simulink model "CarsimOut_1210"  (R2015b)
settings: Solver=VariableStepAuto  StartTime=0.0  StopTime=10.0  RelTol=1e-3
undefined symbols (not defined in the file or in its folder): sigbuilder_block
libraries: Solver_SF x2
settings Model: Creator=ASUS  LastModifiedBy=ASUS

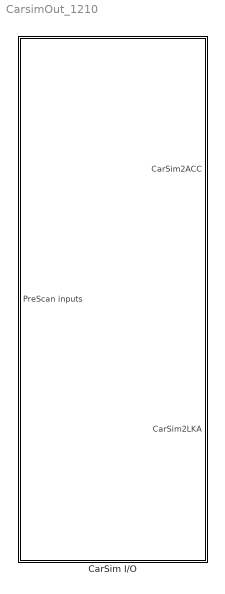
== system CarsimOut_1210 ==
  CarSim I/O : Subsystem

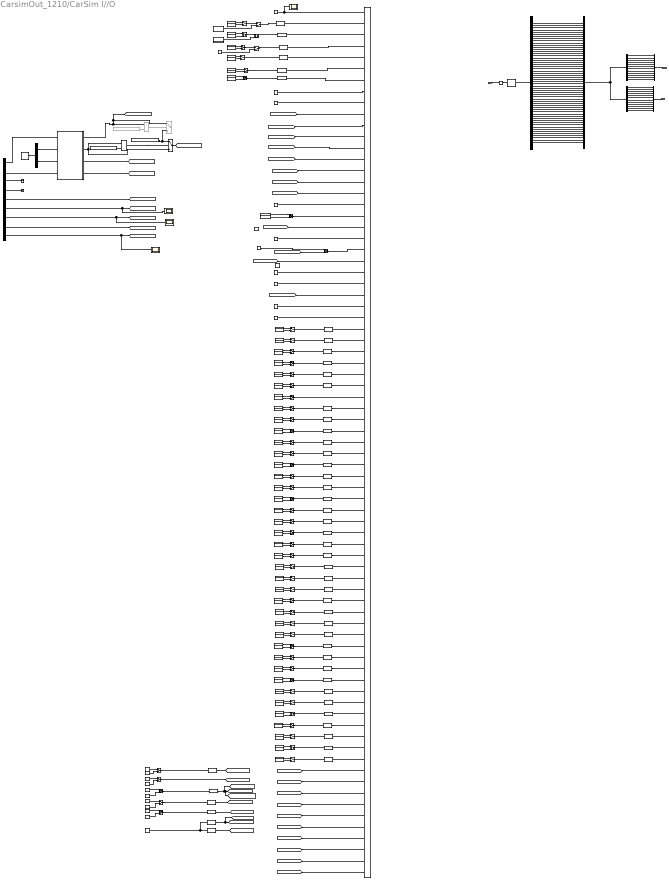
== system CarsimOut_1210/CarSim I//O ==
  PreScan inputs : Inport
  AccelActuPosHSC1_d : Constant  Value=0.31  OutDataTypeStr=double
      settings: AttributesFormatString=%<DataType=%<OutDataTypeStr>>
  BrkPdlPos_H1HSC1_d : Constant  Value=0  OutDataTypeStr=double
  Bus Creator : BusCreator  Inputs=77
  Bus Creator1 : BusCreator  Inputs=56
  Bus Creator2 : BusCreator  Inputs=12
  Bus Creator3 : BusCreator  Inputs=12
  Bus Selector : BusSelector  OutputSignals=EnSpdHSC1_d[rpm] (signal 36),EnToqActuExtdRngHSC1_d[N M] (signal 37),WhlGndVelRDrvn_H1HSC2_d[km/h] (signal 38),WhlGndVelLDrvn_H1HSC2_d[km/h] (signal 39),WhlGndVelRNonDrvn_H1HSC2_d[km/h] (signal 40),WhlGndVelLNonDrvn_H1HSC2_d[km/h] (signal 41),VSELongtAcc_H1HSC1_d[g] (signal 42),VehDynYawRate_H1HSC1_d[deg/s] (signal 43),StrgWhlAngGrd_HSC2_d[deg/s] (signal 44),SteeringWheelAngle[deg] (signal 34),AccelActuPosHSC1_d (signal 45),AccelEfctvPosHSC1_d (signal 46)
  Bus Selector1 : BusSelector  OutputSignals=VehicleCoG_Vx[km/h] (signal 4),Mz_Kp_L1[NM] (signal 48),Mz_Kp_L1[NM] (signal 49),Steer_L1[deg] (signal 50),Steer_R1[deg] (signal 51),F_TRdL1[N] (signal 52),F_TRdR1[N] (signal 53),SteeringWheelAngle[deg] (signal 34),VehDynYawRate_H1HSC1_d[deg/s] (signal 43),Ax_SM[g] (signal 54),Ay_SM[g] (signal 55),GearStatus (signal 56)
  CarSim S-Function2 : Solver_SF/CarSim S-Function2  Priority=1  VehicleCode=i_i  SIMFILE=simfile.sim
      settings: AttributesFormatString=Vehicle Code: %<VehicleCode>
  Carsim Trans Module : Subsystem
  Constant1 : Constant  Value=100
  Constant{2..3,5,8,10,13,16,18,20..21,23,26..27,29,31..32,34,38,40..41,43,45..46,48,52..53,55,58,60..61,63,66,68..69,71,74..75,77,80,82..83,85,88..89} (44 alike) : Constant  Value=0
  Constant{4,6..7,9,11..12,14,17,22,24,28,30,33,35..37,39,42,44,47,49..51,54,56..57,59,62,64..65,67,70,72..73,76,78..79,81,84,86..87,90..91} (43 alike) : Constant
  Constant15 : Constant  OutDataTypeStr=uint8
  Constant19 : Constant  Value=-100
  Constant25 : Constant  Value=300
  DA_IN_DgrObjSyncCtr_u8 : Constant  Value=0  OutDataTypeStr=uint8
  Data Type Conversion{,1..5,10,17,25,32,49,52} (12 alike) : DataTypeConversion  OutDataTypeStr=uint8
  Data Type Conversion{6..8,11..16,18..24,26..31,33..38} (28 alike) : DataTypeConversion
  Data Type Conversion{39..44} (6 alike) : DataTypeConversion  OutDataTypeStr=boolean
  Data Type Conversion{50..51,53..54} (4 alike) : DataTypeConversion  OutDataTypeStr=single
  Demux : Demux  Outputs=56
  Demux1 : Demux  Outputs=[1 3]
  Demux2 : Demux  Outputs=[1 3 1 1 1 1 1 1 1]
  DrvrSbltAtcHSC1_u8 : Constant  OutDataTypeStr=uint8
  EPBAppcnStsHSC1_u8 : Constant  Value=0  OutDataTypeStr=uint8
  EnTypHSC2_u8 : Constant  OutDataTypeStr=uint8
  FntLatDist1 : Constant  Value=3  OutDataTypeStr=double
      settings: AttributesFormatString=%<OutDataTypeStr>
  FntLatDist2 : Constant  Value=0  OutDataTypeStr=double
      settings: AttributesFormatString=%<OutDataTypeStr>
  FntLatDist3 : Constant  OutDataTypeStr=double
      settings: AttributesFormatString=%<OutDataTypeStr>
  FntLatDist4 : Constant  Value=0  OutDataTypeStr=double
      settings: AttributesFormatString=%<OutDataTypeStr>
  FntLatDist5 : Constant  Value=13  OutDataTypeStr=double
      settings: AttributesFormatString=%<OutDataTypeStr>
  FntLatDist6 : Constant  Value=0  OutDataTypeStr=double
      settings: AttributesFormatString=%<OutDataTypeStr>
  ID_LOCKON_u1 : Constant  Value=5  OutDataTypeStr=uint8
  ID_LOCKON_u2 : Constant  Value=0  OutDataTypeStr=uint8
  ID_LOCKON_u3 : Constant  Value=5  OutDataTypeStr=uint8
  ID_LOCKON_u4 : Constant  Value=0  OutDataTypeStr=uint8
  ID_LOCKON_u8 : Constant  Value=5  OutDataTypeStr=uint8
  Lead Car : Solver_SF/CarSim S-Function2  Priority=1  VehicleCode=i_i  SIMFILE=Radar_Acc_ExtSen_Car_1.sim
      settings: AttributesFormatString=Vehicle Code: %<VehicleCode>
  Manual Switch{1,7,11,14,48..49,55} (7 alike) : ManualSwitch  CurrentSetting=0
  Manual Switch{2..6,8..10,12..13,15..47,50..54} (48 alike) : ManualSwitch
  Memory : Memory
  PtBrkPdlDscrtInptStsHSC1_u8 : Constant  Value=0  OutDataTypeStr=uint8
  Pulse Generator : DiscretePulseGenerator  PulseType=Time based  Period=100  PulseWidth=5  PhaseDelay=0.1
  Relational Operator2 : RelationalOperator  Operator=<=  OutDataTypeStr=boolean
  Relational Operator3 : RelationalOperator  Commented=on  Operator=<=  OutDataTypeStr=boolean
  S_ACCAEBTgtLockSts : Scope
  S_ACCAEBTgtLockSts1 : Scope
  S_ACCAEBTgtLockSts2 : Scope
  Signal Builder1 : Subsystem  Tag=STV Subsys  LoadFcn=sigbuilder_block('load');  StartFcn=sigbuilder_block('start');  StopFcn=sigbuilder_block('stop');  ClipboardFcn=sigbuilder_block('clipboard');  mask(Sigbuilder block){}
      mask help: Simulink:masks:SigbuilderBlock_MD
      mask init:
      | if ~strcmp(get_param(bdroot(gcbh),'SimulationStatus'),'stopped') tuvar = sigbuilder_block('maskInit'); end
      settings: CopyFcn=sigbuilder_block('copy');  DeleteFcn=sigbuilder_block('delete');  ModelCloseFcn=sigbuilder_block('modelClose');  PreSaveFcn=sigbuilder_block('preSave');  PauseFcn=sigbuilder_block('pause');  ContinueFcn=sigbuilder_block('continue');  NameChangeFcn=sigbuilder_block('namechange');  OpenFcn=sigbuilder_block('open',[437.6 199.2 550.4 400 ]);  CloseFcn=sigbuilder_block('close');
      mask Display: plot(0, 0, 100, 100,[2, 2, 32, 32, 2], [68, 8, 8, 68, 68],[32, 2], [38, 38], [32, 19, 2],[53, 60, 44], [32, 17, 17, 2],[16, 16, 31, 31]);txt = getActiveGroup(gcbh);text(2, 100, txt,'verticalAlignment', 'top');
  Signal Builder2 : Subsystem  Tag=STV Subsys  LoadFcn=sigbuilder_block('load');  StartFcn=sigbuilder_block('start');  StopFcn=sigbuilder_block('stop');  ClipboardFcn=sigbuilder_block('clipboard');  mask(Sigbuilder block){}
      mask help: Simulink:masks:SigbuilderBlock_MD
      mask init:
      | if ~strcmp(get_param(bdroot(gcbh),'SimulationStatus'),'stopped') tuvar = sigbuilder_block('maskInit'); end
      settings: CopyFcn=sigbuilder_block('copy');  DeleteFcn=sigbuilder_block('delete');  ModelCloseFcn=sigbuilder_block('modelClose');  PreSaveFcn=sigbuilder_block('preSave');  PauseFcn=sigbuilder_block('pause');  ContinueFcn=sigbuilder_block('continue');  NameChangeFcn=sigbuilder_block('namechange');  OpenFcn=sigbuilder_block('open',[437.6 199.2 550.4 400 ]);  CloseFcn=sigbuilder_block('close');
      mask Display: plot(0, 0, 100, 100,[2, 2, 32, 32, 2], [68, 8, 8, 68, 68],[32, 2], [38, 38], [32, 19, 2],[53, 60, 44], [32, 17, 17, 2],[16, 16, 31, 31]);txt = getActiveGroup(gcbh);text(2, 100, txt,'verticalAlignment', 'top');
  StrgWhlAngGrd_HSC2_d : Constant  Value=0  OutDataTypeStr=double
  StrgWhlAngHSC2_d : Constant  OutDataTypeStr=double
      settings: AttributesFormatString=%<DataType=%<OutDataTypeStr>>
  Switch : Switch  Criteria=u2 ~= 0
  Switch1 : Switch  Commented=on  Criteria=u2 ~= 0
  SysPwrMd_H1HSC1_u8 : Constant  Value=3  OutDataTypeStr=uint8
      settings: AttributesFormatString=%<DataType=%<OutDataTypeStr>>
  Terminator1 : Terminator
  Terminator3 : Terminator
  TrEstdGear_HSC1_u8 : Constant  Value=4  OutDataTypeStr=uint8
  TrShftLvrPosHSC1_u8 : Constant  Value=4  OutDataTypeStr=uint8
  VSELongtAcc_H1HSC1_d : Scope
  VehDynYawRate_H1HSC1_d : Constant  Value=10  OutDataTypeStr=double
  const_2 : Constant  Description=Cancel the Integral work performance  Value=0.02  OutDataTypeStr=single
      settings: AttributesFormatString=|
      | %<Description>
      | %<OutDataTypeStr>
  const_3 : Constant  Description=Cancel the Integral work performance  Value=0  OutDataTypeStr=single
      settings: AttributesFormatString=|
      | %<Description>
      | %<OutDataTypeStr>
  const_5 : Constant  Description=Cancel the Integral work performance  Commented=on  Value=-0.02  OutDataTypeStr=single
      settings: AttributesFormatString=|
      | %<Description>
      | %<OutDataTypeStr>
  CarSim2ACC : Outport
  CarSim2LKA : Outport  Port=2
  wires:
  ? -> Demux2/1
  Lead Car/1 -> Demux1/1
  Demux1/2 -> Carsim Trans Module/3(Rd_Hd_Veh_Data)
  Demux2/2 -> Carsim Trans Module/4(Follow_Vehicle_Data)
  Demux2/1 -> Carsim Trans Module/1(Follow_Vehicle_Spd)  "FL_veh_spd"
  Demux2/4 -> Terminator1/1  "AT_Gear"
  Demux2/5 -> [EnSpdHSC1_d]  "EnSpdHSC1_d"
  Demux1/1 -> Carsim Trans Module/2(Hd_Vehicle_Spd)
  Demux2/3 -> Terminator3/1  "StrWhlAngRt"
  Carsim Trans Module/2(AvgVehSpd) -> Switch/3, Relational Operator2/1  "AvgVehSpd_NF"
  Carsim Trans Module/4("Lateral_Distance ") -> [X_POSITION_LOCKON_d]
  Demux2/7 -> VSELongtAcc_H1HSC1_d/1, [VSELongtAcc_H1HSC1_d]  "VSELongtAcc_H1HSC1_d"
  Demux2/6 -> S_ACCAEBTgtLockSts2/1, [AccelActuPosHSC1_d]  "AccelActuPosHSC1_d"
  TrEstdGear_HSC1_u8/1 -> Bus Creator/24  "TrEstdGear_HSC1_u8"
  [StrAngDriver_d] -> Bus Creator/20  "StrgWhlAngGrd_HSC2_d"
  [VELOCITY_LOCKON_d] -> Bus Creator/10  "VELOCITY_LOCKON_d"
  [X_POSITION_LOCKON_d] -> Bus Creator/15  "X_POSITION_LOCKON_d"
  [VehDynYawRate_H1HSC1_d] -> Bus Creator/23  "VehDynYawRate_H1HSC1_d"
  ID_LOCKON_u8/1 -> S_ACCAEBTgtLockSts/1, Bus Creator/1  "ID_LOCKON_u8"
  Manual Switch8/1 -> Bus Creator/19  "PtBrkPdlDscrtInptStsHSC1_u8"
  BrkPdlPos_H1HSC1_d/1 -> Bus Creator/18  "BrkPdlPos_H1HSC1_d"
  TrShftLvrPosHSC1_u8/1 -> Bus Creator/9  "TrShftLvrPosHSC1_u8"
  EnTypHSC2_u8/1 -> Bus Creator/25  "EnTypHSC2_u8"
  DrvrSbltAtcHSC1_u8/1 -> Bus Creator/27  "DrvrSbltAtcHSC1_u8"
  EPBAppcnStsHSC1_u8/1 -> Bus Creator/28  "EPBAppcnStsHSC1_u8"
  SysPwrMd_H1HSC1_u8/1 -> Bus Creator/8  "SysPwrMd_H1HSC1_u8"
  [VSELongtAcc_H1HSC1_d] -> Bus Creator/17  "VSELongtAcc_H1HSC1_d"
  StrgWhlAngHSC2_d/1 -> Bus Creator/21  "StrgWhlAngHSC2_d"
  [WhlGndVelRDrvn_H1HSC2_d] -> Bus Creator/11  "WhlGndVelRDrvn_H1HSC2_d"
  [WhlGndVelRDrvn_H1HSC2_d] -> Bus Creator/12  "WhlGndVelLDrvn_H1HSC2_d"
  [WhlGndVelRDrvn_H1HSC2_d] -> Bus Creator/13  "WhlGndVelRNonDrvn_H1HSC2_d"
  [WhlGndVelRDrvn_H1HSC2_d] -> Bus Creator/14  "WhlGndVelLNonDrvn_H1HSC2_d"
  Manual Switch48/1 -> Data Type Conversion1/1  "CCSwStsSpdDecSwAHSC1_u8"
  Manual Switch1/1 -> Data Type Conversion4/1  "CCSwStsOnSwAHSC1_u8"
  Manual Switch2/1 -> Data Type Conversion5/1  "CCSwStsCanclSwAHSC1_u8"
  Manual Switch49/1 -> Data Type Conversion2/1  "CCSwStsSetSwAHSC1_u8"
  Manual Switch55/1 -> Data Type Conversion/1  "CCSwStsSpdIncSwAHSC1_u8"
  Manual Switch3/1 -> Data Type Conversion3/1  "CCSwStsRsmSwAHSC1_u8"
  Constant4/1 -> Manual Switch2/2
  Constant3/1 -> Manual Switch2/1
  Constant7/1 -> Manual Switch3/2
  Constant5/1 -> Manual Switch3/1
  Constant9/1 -> Manual Switch4/2
  Constant8/1 -> Manual Switch4/1
  Constant14/1 -> Manual Switch5/2
  Constant13/1 -> Manual Switch5/1
  Constant11/1 -> Manual Switch6/2
  Constant10/1 -> Manual Switch6/1
  Constant12/1 -> Manual Switch1/2
  Constant2/1 -> Manual Switch1/1
  Carsim Trans Module/3(Longt_Distance) -> [Y_POSITION_LOCKON_d]
  [EnSpdHSC1_d] -> Bus Creator/26  "EnSpdHSC1_d"
  [Y_POSITION_LOCKON_d] -> Bus Creator/16  "Y_POSITION_LOCKON_d"
  [AccelActuPosHSC1_d] -> Manual Switch7/2
  Data Type Conversion/1 -> Bus Creator/2  "CCSwStsSpdIncSwAHSC1_u8"
  Data Type Conversion1/1 -> Bus Creator/3  "CCSwStsSpdDecSwAHSC1_u8"
  Data Type Conversion2/1 -> Bus Creator/4  "CCSwStsSetSwAHSC1_u8"
  Data Type Conversion3/1 -> Bus Creator/5  "CCSwStsRsmSwAHSC1_u8"
  Data Type Conversion4/1 -> Bus Creator/6  "CCSwStsOnSwAHSC1_u8"
  Data Type Conversion5/1 -> Bus Creator/7  "CCSwStsCanclSwAHSC1_u8"
  PtBrkPdlDscrtInptStsHSC1_u8/1 -> Manual Switch8/1  "PtBrkPdlDscrtInptStsHSC1_u8"
  Constant15/1 -> Manual Switch8/2
  Manual Switch7/1 -> Bus Creator/22  "AccelActuPosHSC1_d"
  AccelActuPosHSC1_d/1 -> Manual Switch7/1
  Demux2/8 -> [StrAngDriver_d]  "StrgWhlAngGrd_HSC2_d"
  Demux2/9 -> S_ACCAEBTgtLockSts1/1, [VehDynYawRate_H1HSC1_d]
  Manual Switch9/1 -> Data Type Conversion18/1
  Constant6/1 -> Manual Switch9/2
  Constant1/1 -> Manual Switch9/1
  Data Type Conversion18/1 -> Bus Creator/31  "EnToqActuExtdRngHSC1_d"
  Manual Switch10/1 -> Data Type Conversion6/1
  Constant17/1 -> Manual Switch10/2
  Constant16/1 -> Manual Switch10/1
  Data Type Conversion6/1 -> Bus Creator/32  "EnToqDrvrReqdExtdRngHSC1_d"
  Manual Switch11/1 -> Data Type Conversion7/1
  Constant19/1 -> Manual Switch11/2
  Constant18/1 -> Manual Switch11/1
  Data Type Conversion7/1 -> Bus Creator/33  "EnToqMinExtdRngHSC1_d"
  Manual Switch14/1 -> Data Type Conversion8/1
  Constant25/1 -> Manual Switch14/2
  Constant20/1 -> Manual Switch14/1
  Data Type Conversion8/1 -> Bus Creator/34  "EnToqMaxExtdRngHSC1_d"
  Constant22/1 -> Manual Switch12/2
  Constant21/1 -> Manual Switch12/1
  Manual Switch12/1 -> Bus Creator/35  "AccelEfctvPosHSC1_d"
  Manual Switch13/1 -> Data Type Conversion10/1
  Constant24/1 -> Manual Switch13/2
  Constant23/1 -> Manual Switch13/1
  Data Type Conversion10/1 -> Bus Creator/36  "Lane0_Lane_Mark_Quality"
  Manual Switch20/1 -> Data Type Conversion11/1
  Constant37/1 -> Manual Switch20/2
  Constant26/1 -> Manual Switch20/1
  Data Type Conversion11/1 -> Bus Creator/37  "Lane0_Lane_View_Range_Start"
  Manual Switch15/1 -> Data Type Conversion12/1
  Constant28/1 -> Manual Switch15/2
  Constant27/1 -> Manual Switch15/1
  Data Type Conversion12/1 -> Bus Creator/38  "Lane0_Lane_View_Range_End"
  Manual Switch16/1 -> Data Type Conversion13/1
  Constant30/1 -> Manual Switch16/2
  Constant29/1 -> Manual Switch16/1
  Data Type Conversion13/1 -> Bus Creator/39  "Lane0_C0_Lane_Position"
  Manual Switch19/1 -> Data Type Conversion14/1
  Constant36/1 -> Manual Switch19/2
  Constant31/1 -> Manual Switch19/1
  Data Type Conversion14/1 -> Bus Creator/40  "Lane0_C1_Heading_Angle"
  Manual Switch17/1 -> Data Type Conversion15/1
  Constant33/1 -> Manual Switch17/2
  Constant32/1 -> Manual Switch17/1
  Data Type Conversion15/1 -> Bus Creator/41  "Lane0_C2_Lane_Curvature"
  Manual Switch18/1 -> Data Type Conversion16/1
  Constant35/1 -> Manual Switch18/2
  Constant34/1 -> Manual Switch18/1
  Data Type Conversion16/1 -> Bus Creator/42  "Lane0_C3_Lane_Curvature_Driv"
  Manual Switch21/1 -> Data Type Conversion17/1
  Constant39/1 -> Manual Switch21/2
  Constant38/1 -> Manual Switch21/1
  Data Type Conversion17/1 -> Bus Creator/43  "Lane1_Lane_Mark_Quality"
  Manual Switch27/1 -> Data Type Conversion19/1
  Constant51/1 -> Manual Switch27/2
  Constant40/1 -> Manual Switch27/1
  Data Type Conversion19/1 -> Bus Creator/44  "Lane1_Lane_View_Range_Start"
  Manual Switch22/1 -> Data Type Conversion20/1
  Constant42/1 -> Manual Switch22/2
  Constant41/1 -> Manual Switch22/1
  Data Type Conversion20/1 -> Bus Creator/45  "Lane1_Lane_View_Range_End"
  Manual Switch23/1 -> Data Type Conversion21/1
  Constant44/1 -> Manual Switch23/2
  Constant43/1 -> Manual Switch23/1
  Data Type Conversion21/1 -> Bus Creator/46  "Lane1_C0_Lane_Position"
  Manual Switch26/1 -> Data Type Conversion22/1
  Constant50/1 -> Manual Switch26/2
  Constant45/1 -> Manual Switch26/1
  Data Type Conversion22/1 -> Bus Creator/47  "Lane1_C1_Heading_Angle"
  Manual Switch24/1 -> Data Type Conversion23/1
  Constant47/1 -> Manual Switch24/2
  Constant46/1 -> Manual Switch24/1
  Data Type Conversion23/1 -> Bus Creator/48  "Lane1_C2_Lane_Curvature"
  Manual Switch25/1 -> Data Type Conversion24/1
  Constant49/1 -> Manual Switch25/2
  Constant48/1 -> Manual Switch25/1
  Data Type Conversion24/1 -> Bus Creator/49  "Lane1_C3_Lane_Curvature_Driv"
  Manual Switch30/1 -> Data Type Conversion25/1
  Constant57/1 -> Manual Switch30/2
  Constant52/1 -> Manual Switch30/1
  Data Type Conversion25/1 -> Bus Creator/50  "Lane2_Lane_Mark_Quality"
  Manual Switch28/1 -> Data Type Conversion26/1
  Constant54/1 -> Manual Switch28/2
  Constant53/1 -> Manual Switch28/1
  Data Type Conversion26/1 -> Bus Creator/51  "Lane2_Lane_View_Range_Start"
  Manual Switch29/1 -> Data Type Conversion27/1
  Constant56/1 -> Manual Switch29/2
  Constant55/1 -> Manual Switch29/1
  Data Type Conversion27/1 -> Bus Creator/52  "Lane2_Lane_View_Range_End"
  Manual Switch31/1 -> Data Type Conversion28/1
  Constant59/1 -> Manual Switch31/2
  Constant58/1 -> Manual Switch31/1
  Data Type Conversion28/1 -> Bus Creator/53  "Lane2_C0_Lane_Position"
  Manual Switch34/1 -> Data Type Conversion29/1
  Constant65/1 -> Manual Switch34/2
  Constant60/1 -> Manual Switch34/1
  Data Type Conversion29/1 -> Bus Creator/54  "Lane2_C1_Heading_Angle"
  Manual Switch32/1 -> Data Type Conversion30/1
  Constant62/1 -> Manual Switch32/2
  Constant61/1 -> Manual Switch32/1
  Data Type Conversion30/1 -> Bus Creator/55  "Lane2_C2_Lane_Curvature"
  Manual Switch33/1 -> Data Type Conversion31/1
  Constant64/1 -> Manual Switch33/2
  Constant63/1 -> Manual Switch33/1
  Data Type Conversion31/1 -> Bus Creator/56  "Lane2_C3_Lane_Curvature_Driv"
  Manual Switch35/1 -> Data Type Conversion32/1
  Constant67/1 -> Manual Switch35/2
  Constant66/1 -> Manual Switch35/1
  Manual Switch38/1 -> Data Type Conversion33/1
  Constant73/1 -> Manual Switch38/2
  Constant68/1 -> Manual Switch38/1
  Manual Switch36/1 -> Data Type Conversion34/1
  Constant70/1 -> Manual Switch36/2
  Constant69/1 -> Manual Switch36/1
  Manual Switch37/1 -> Data Type Conversion35/1
  Constant72/1 -> Manual Switch37/2
  Constant71/1 -> Manual Switch37/1
  Manual Switch41/1 -> Data Type Conversion36/1
  Constant79/1 -> Manual Switch41/2
  Constant74/1 -> Manual Switch41/1
  Manual Switch39/1 -> Data Type Conversion37/1
  Constant76/1 -> Manual Switch39/2
  Constant75/1 -> Manual Switch39/1
  Manual Switch40/1 -> Data Type Conversion38/1
  Constant78/1 -> Manual Switch40/2
  Constant77/1 -> Manual Switch40/1
  Manual Switch42/1 -> Data Type Conversion39/1
  Constant81/1 -> Manual Switch42/2
  Constant80/1 -> Manual Switch42/1
  Manual Switch45/1 -> Data Type Conversion40/1
  Constant87/1 -> Manual Switch45/2
  Constant82/1 -> Manual Switch45/1
  Manual Switch43/1 -> Data Type Conversion41/1
  Constant84/1 -> Manual Switch43/2
  Constant83/1 -> Manual Switch43/1
  Manual Switch44/1 -> Data Type Conversion42/1
  Constant86/1 -> Manual Switch44/2
  Constant85/1 -> Manual Switch44/1
  Data Type Conversion37/1 -> Bus Creator/62  "Lane3_C2_Lane_Curvature"
  Data Type Conversion42/1 -> Bus Creator/67  "MainBeamLghtOnHSC1"
  Data Type Conversion38/1 -> Bus Creator/63  "Lane3_C3_Lane_Curvature_Driv"
  Data Type Conversion40/1 -> Bus Creator/65  "FrtFogLghtOnHSC1"
  Data Type Conversion36/1 -> Bus Creator/61  "Lane3_C1_Heading_Angle"
  Data Type Conversion41/1 -> Bus Creator/66  "DipdBeamLghtOnHSC1"
  Data Type Conversion39/1 -> Bus Creator/64  "RrFogLghtOnHSC1_b"
  Data Type Conversion34/1 -> Bus Creator/59  "Lane3_Lane_View_Range_End"
  Data Type Conversion35/1 -> Bus Creator/60  "Lane3_C0_Lane_Position"
  Data Type Conversion32/1 -> Bus Creator/57  "Lane3_Lane_Mark_Quality"
  Data Type Conversion33/1 -> Bus Creator/58  "Lane3_Lane_View_Range_Start"
  Manual Switch47/1 -> Data Type Conversion43/1
  Constant91/1 -> Manual Switch47/2
  Constant88/1 -> Manual Switch47/1
  Data Type Conversion43/1 -> Bus Creator/29  "RDircnIOHSC1_b"
  Manual Switch46/1 -> Data Type Conversion44/1
  Constant90/1 -> Manual Switch46/2
  Constant89/1 -> Manual Switch46/1
  Data Type Conversion44/1 -> Bus Creator/30  "LDircnIOHSC1_b"
  const_2/1 -> Relational Operator2/2
  Relational Operator2/1 -> Switch/2
  const_3/1 -> Switch1/3, Switch/1
  Switch/1 -> [WhlGndVelRDrvn_H1HSC2_d]
  Carsim Trans Module/1(Relative Speed) -> [VELOCITY_LOCKON_d], Switch1/1, Relational Operator3/1
  const_5/1 -> Relational Operator3/2
  Relational Operator3/1 -> Switch1/2
  Manual Switch6/1 -> Manual Switch48/1  "CCSwStsSpdDecSwAHSC1_u8"
  Pulse Generator/1 -> Manual Switch49/2
  Manual Switch4/1 -> Manual Switch49/1
  [DA_IN_indx_RCARrTgtID_u8] -> Bus Creator/68  "DA_IN_indx_RCARrTgtID_u8"
  [DA_IN_v_RMRltVehSpd_sg] -> Bus Creator/69  "DA_IN_v_RMRltVehSpd_sg"
  [DA_IN_d_RMRdrLongtDist_sg] -> Bus Creator/71  "DA_IN_d_RMRdrLongtDist_sg"
  [DA_IN_DgrObjId_u8] -> Bus Creator/72  "DA_IN_DgrObjId_u8"
  [DA_IN_DgrObjLatRltvDist_sg] -> Bus Creator/73  "DA_IN_DgrObjLatRltvDist_sg"
  [DA_IN_DgrObjLatRltvSpd_sg] -> Bus Creator/74  "DA_IN_DgrObjLatRltvSpd_sg"
  [DA_IN_DgrObjLongtRltvSpd_sg] -> Bus Creator/77  "DA_IN_DgrObjLongtRltvSpd_sg"
  [DA_IN_DgrObjLongtRltvDist_sg] -> Bus Creator/75  "DA_IN_DgrObjLongtRltvDist_sg"
  [DA_IN_DgrObjSyncCtr_u8] -> Bus Creator/76  "DA_IN_DgrObjSyncCtr_u8"
  [DA_IN_d_RMRdrLatDist_sg] -> Bus Creator/70  "DA_IN_d_RMRdrLatDist_sg"
  ID_LOCKON_u1/1 -> Manual Switch50/1
  ID_LOCKON_u2/1 -> Manual Switch50/2
  Manual Switch50/1 -> Data Type Conversion49/1
  ID_LOCKON_u3/1 -> Manual Switch51/1
  ID_LOCKON_u4/1 -> Manual Switch51/2
  Manual Switch51/1 -> [DA_IN_indx_RCARrTgtID_u8]
  Data Type Conversion49/1 -> [DA_IN_DgrObjId_u8]
  FntLatDist5/1 -> Manual Switch52/1
  FntLatDist6/1 -> Manual Switch52/2
  Manual Switch52/1 -> Data Type Conversion51/1
  FntLatDist3/1 -> Manual Switch53/1
  FntLatDist4/1 -> Manual Switch53/2
  Manual Switch53/1 -> Data Type Conversion50/1
  FntLatDist1/1 -> Manual Switch54/1
  FntLatDist2/1 -> Manual Switch54/2
  Manual Switch54/1 -> Data Type Conversion53/1
  DA_IN_DgrObjSyncCtr_u8/1 -> Data Type Conversion52/1, Data Type Conversion54/1
  Data Type Conversion50/1 -> [DA_IN_DgrObjLatRltvDist_sg]
  Data Type Conversion51/1 -> [DA_IN_d_RMRdrLongtDist_sg], [DA_IN_d_RMRdrLatDist_sg], [DA_IN_DgrObjLongtRltvDist_sg]
  Data Type Conversion52/1 -> [DA_IN_DgrObjSyncCtr_u8]
  Data Type Conversion53/1 -> [DA_IN_DgrObjLongtRltvSpd_sg]
  Data Type Conversion54/1 -> [DA_IN_v_RMRltVehSpd_sg], [DA_IN_DgrObjLatRltvSpd_sg]
  Manual Switch5/1 -> Manual Switch55/1  "CCSwStsSpdIncSwAHSC1_u8"
  Signal Builder1/1(Signal 1) -> Manual Switch55/2
  Signal Builder2/1(Signal 1) -> Manual Switch48/2
  CarSim S-Function2/1 -> Demux/1
  PreScan inputs/1 -> Memory/1
  Memory/1 -> CarSim S-Function2/1
  Demux/13 -> Bus Creator1/13  "CarSim_Pos_Wheel_FR_x[m]"
  Demux/6 -> Bus Creator1/6  "VehicleCoG_Vz[km/h]"
  Demux/11 -> Bus Creator1/11  "CarSim_Pos_Wheel_FL_y[m]"
  Demux/12 -> Bus Creator1/12  "CarSim_Pos_Wheel_FL_z[m]"
  Demux/2 -> Bus Creator1/2  "SprungMass_Pos_Global_y[m]"
  Demux/14 -> Bus Creator1/14  "CarSim_Pos_Wheel_FR_y[m]"
  Demux/15 -> Bus Creator1/15  "CarSim_Pos_Wheel_FR_z[m]"
  Demux/1 -> Bus Creator1/1  "SprungMass_Pos_Global_x[m]"
  Demux/16 -> Bus Creator1/16  "CarSim_Pos_Wheel_RL_x[m]"
  Demux/17 -> Bus Creator1/17  "CarSim_Pos_Wheel_RL_y[m]"
  Demux/4 -> Bus Creator1/4  "VehicleCoG_Vx[km/h]"
  Demux/3 -> Bus Creator1/3  "SprungMass_Pos_Global_z[m]"
  Demux/7 -> Bus Creator1/7  "SprungMass_Angle_Global_Roll[deg]"
  Demux/8 -> Bus Creator1/8  "SprungMass_Angle_Global_Pitch[deg]"
  Demux/9 -> Bus Creator1/9  "SprungMass_Angle_Global_Yaw[deg]"
  Demux/10 -> Bus Creator1/10  "CarSim_Pos_Wheel_FL_x[m]"
  Demux/5 -> Bus Creator1/5  "VehicleCoG_Vy[km/h]"
  Demux/20 -> Bus Creator1/20  "CarSim_Pos_Wheel_RR_y[m]"
  Demux/19 -> Bus Creator1/19  "CarSim_Pos_Wheel_RR_x[m]"
  Demux/18 -> Bus Creator1/18  "CarSim_Pos_Wheel_RL_Z[m]"
  Demux/28 -> Bus Creator1/28  "CarSim_Angle_Wheel_RL_Roll[deg]"
  Demux/30 -> Bus Creator1/30  "CarSim_Angle_Wheel_RL_Steer[deg]"
  Demux/22 -> Bus Creator1/22  "CarSim_Angle_Wheel_FL_Roll[deg]"
  Demux/21 -> Bus Creator1/21  "CarSim_Pos_Wheel_RR_z[m]"
  Demux/27 -> Bus Creator1/27  "CarSim_Angle_Wheel_FR_Steer[deg]"
  Demux/29 -> Bus Creator1/29  "CarSim_Angle_Wheel_RL_Rot[rev]"
  Demux/24 -> Bus Creator1/24  "CarSim_Angle_Wheel_FL_Steer[deg]"
  Demux/23 -> Bus Creator1/23  "CarSim_Angle_Wheel_FL_Rot[rev]"
  Demux/26 -> Bus Creator1/26  "CarSim_Angle_Wheel_FR_Rot[rev]"
  Demux/25 -> Bus Creator1/25  "CarSim_Angle_Wheel_FR_Roll[deg]"
  Bus Creator1/1 -> Bus Selector/1, Bus Selector1/1
  Demux/31 -> Bus Creator1/31  "CarSim_Angle_Wheel_RR_Roll[deg]"
  Demux/32 -> Bus Creator1/32  "CarSim_Angle_Wheel_RR_Rot[rev]"
  Demux/33 -> Bus Creator1/33  "CarSim_Angle_Wheel_RR_Steer[deg]"
  Demux/34 -> Bus Creator1/34  "SteeringWheelAngle[deg]"
  Demux/35 -> Bus Creator1/35  "Axle1ReducedSW"
  Demux/36 -> Bus Creator1/36  "EnSpdHSC1_d[rpm]"
  Demux/37 -> Bus Creator1/37  "EnToqActuExtdRngHSC1_d[N M]"
  Demux/38 -> Bus Creator1/38  "WhlGndVelRDrvn_H1HSC2_d[km/h]"
  Demux/39 -> Bus Creator1/39  "WhlGndVelLDrvn_H1HSC2_d[km/h]"
  Demux/40 -> Bus Creator1/40  "WhlGndVelRNonDrvn_H1HSC2_d[km/h]"
  Demux/41 -> Bus Creator1/41  "WhlGndVelLNonDrvn_H1HSC2_d[km/h]"
  Demux/42 -> Bus Creator1/42  "VSELongtAcc_H1HSC1_d[g]"
  Demux/43 -> Bus Creator1/43  "VehDynYawRate_H1HSC1_d[deg/s]"
  Demux/44 -> Bus Creator1/44  "StrgWhlAngGrd_HSC2_d[deg/s]"
  Demux/45 -> Bus Creator1/45  "AccelActuPosHSC1_d"
  Demux/46 -> Bus Creator1/46  "AccelEfctvPosHSC1_d"
  Demux/47 -> Bus Creator1/47  "Pbk_Con[MPa]"
  Demux/48 -> Bus Creator1/48  "Mz_Kp_L1[NM]"
  Demux/49 -> Bus Creator1/49  "Mz_Kp_L1[NM]"
  Demux/50 -> Bus Creator1/50  "Steer_L1[deg]"
  Demux/51 -> Bus Creator1/51  "Steer_R1[deg]"
  Demux/52 -> Bus Creator1/52  "F_TRdL1[N]"
  Demux/53 -> Bus Creator1/53  "F_TRdR1[N]"
  Demux/54 -> Bus Creator1/54  "Ax_SM[g]"
  Demux/55 -> Bus Creator1/55  "Ay_SM[g]"
  Demux/56 -> Bus Creator1/56  "GearStatus"
  Bus Selector1/8 -> Bus Creator2/8  "<SteeringWheelAngle[deg] (signal 34)>"
  Bus Selector1/9 -> Bus Creator2/9  "<VehDynYawRate_H1HSC1_d[deg/s] (signal 43)>"
  Bus Selector1/11 -> Bus Creator2/11  "<Ay_SM[g] (signal 55)>"
  Bus Selector1/10 -> Bus Creator2/10  "<Ax_SM[g] (signal 54)>"
  Bus Selector1/12 -> Bus Creator2/12  "<GearStatus (signal 56)>"
  Bus Selector1/2 -> Bus Creator2/2  "<Mz_Kp_L1[NM] (signal 48)>"
  Bus Selector1/4 -> Bus Creator2/4  "<Steer_L1[deg] (signal 50)>"
  Bus Selector1/5 -> Bus Creator2/5  "<Steer_R1[deg] (signal 51)>"
  Bus Selector1/6 -> Bus Creator2/6  "<F_TRdL1[N] (signal 52)>"
  Bus Selector1/7 -> Bus Creator2/7  "<F_TRdR1[N] (signal 53)>"
  Bus Selector1/1 -> Bus Creator2/1  "<VehicleCoG_Vx[km/h] (signal 4)>"
  Bus Selector1/3 -> Bus Creator2/3  "<Mz_Kp_L1[NM] (signal 49)>"
  Bus Creator2/1 -> CarSim2LKA/1
  Bus Selector/1 -> Bus Creator3/1  "<EnSpdHSC1_d[rpm] (signal 36)>"
  Bus Selector/2 -> Bus Creator3/2  "<EnToqActuExtdRngHSC1_d[N M] (signal 37)>"
  Bus Selector/3 -> Bus Creator3/3  "<WhlGndVelRDrvn_H1HSC2_d[km/h] (signal 38)>"
  Bus Selector/4 -> Bus Creator3/4  "<WhlGndVelLDrvn_H1HSC2_d[km/h] (signal 39)>"
  Bus Selector/5 -> Bus Creator3/5  "<WhlGndVelRNonDrvn_H1HSC2_d[km/h] (signal 40)>"
  Bus Selector/6 -> Bus Creator3/6  "<WhlGndVelLNonDrvn_H1HSC2_d[km/h] (signal 41)>"
  Bus Selector/7 -> Bus Creator3/7  "<VSELongtAcc_H1HSC1_d[g] (signal 42)>"
  Bus Selector/8 -> Bus Creator3/8  "<VehDynYawRate_H1HSC1_d[deg/s] (signal 43)>"
  Bus Selector/9 -> Bus Creator3/9  "<StrgWhlAngGrd_HSC2_d[deg/s] (signal 44)>"
  Bus Selector/10 -> Bus Creator3/10  "<SteeringWheelAngle[deg] (signal 34)>"
  Bus Selector/11 -> Bus Creator3/11  "<AccelActuPosHSC1_d (signal 45)>"
  Bus Selector/12 -> Bus Creator3/12  "<AccelEfctvPosHSC1_d (signal 46)>"
  Bus Creator3/1 -> CarSim2ACC/1

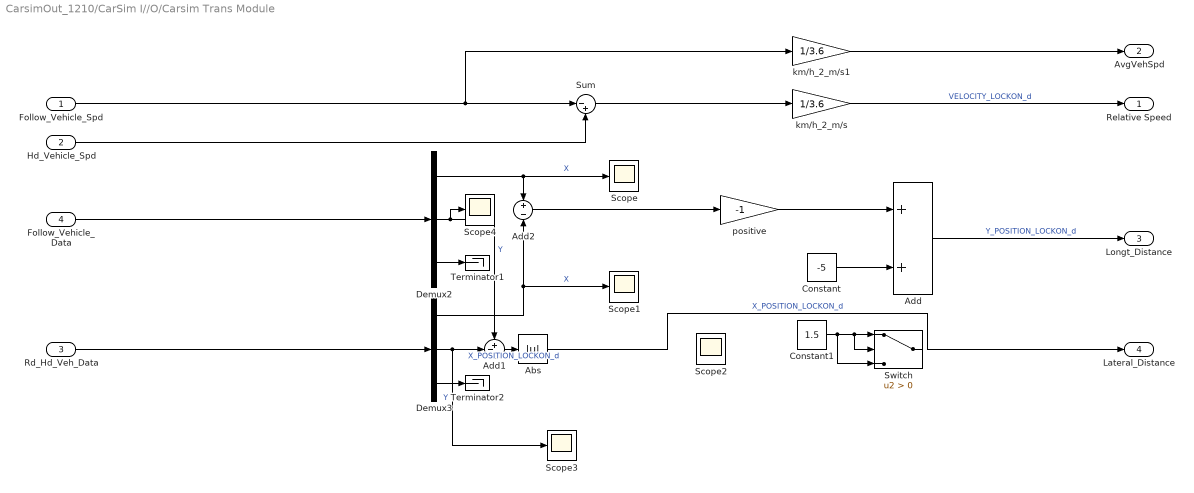
== system CarsimOut_1210/CarSim I//O/Carsim Trans Module ==
  Follow_Vehicle_Spd : Inport
  Hd_Vehicle_Spd : Inport  Port=2
  Rd_Hd_Veh_Data : Inport  Port=3
  Follow_Vehicle_Data : Inport  Port=4
  Abs : Abs
  Add : Sum
  Add1 : Sum  Inputs=+-|
  Add2 : Sum  Inputs=+-
  Constant : Constant  Value=-5
  Constant1 : Constant  Value=1.5
  Demux2 : Demux  Outputs=3
  Demux3 : Demux  Outputs=3
  Scope{,1..4} (5 alike) : Scope
  Sum : Sum  Inputs=|-+
  Switch : Switch  Criteria=u2 > Threshold
  Terminator1 : Terminator
  Terminator2 : Terminator
  km/h_2_m/s : Gain  Gain=1/3.6
  km/h_2_m/s1 : Gain  Gain=1/3.6
  positive : Gain  Gain=-1
  Relative Speed : Outport
  AvgVehSpd : Outport  Port=2
  Longt_Distance : Outport  Port=3
  "Lateral_Distance " : Outport  Port=4
  wires:
  Rd_Hd_Veh_Data/1 -> Demux3/1
  Follow_Vehicle_Data/1 -> Demux2/1
  Demux2/3 -> Terminator1/1
  Hd_Vehicle_Spd/1 -> Sum/2
  Demux3/3 -> Terminator2/1
  Demux3/1 -> Scope1/1, Add2/2  "X"
  Demux2/1 -> Add2/1, Scope/1  "X"
  Demux3/2 -> Scope3/1, Add1/2  "Y"
  Demux2/2 -> Scope4/1, Add1/1  "Y"
  Follow_Vehicle_Spd/1 -> km/h_2_m/s1/1, Sum/1
  Sum/1 -> km/h_2_m/s/1
  Add2/1 -> positive/1
  km/h_2_m/s/1 -> Relative Speed/1  "VELOCITY_LOCKON_d"
  positive/1 -> Add/1
  km/h_2_m/s1/1 -> AvgVehSpd/1
  Add/1 -> Longt_Distance/1  "Y_POSITION_LOCKON_d"
  Constant/1 -> Add/2
  Abs/1 -> "Lateral_Distance "/1  "X_POSITION_LOCKON_d"
  Constant1/1 -> Switch/3, Switch/2, Switch/1
  Add1/1 -> Abs/1  "X_POSITION_LOCKON_d"

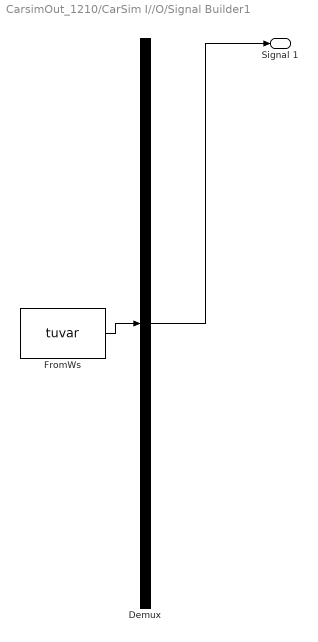
== system CarsimOut_1210/CarSim I//O/Signal Builder1 ==
  Demux : Demux  Tag=STV Demux  Outputs=1
  FromWs : FromWorkspace  Tag=STV FromWs  VariableName=tuvar  SampleTime=0
      SigBuilderData=|
      | common.afterFinalStr = 'Extrapolate'
      | common.sampleTime = 0
      | dataSet.timeRange = [0 10]
      | dataSet.name = 'Group 1'
      | sbobj.Groups.Name = 'Group 1'
      | sbobj.Groups.Signals.Name = 'Signal 1'
      | sbobj.Groups.Signals.XData = [0 1 1 1.003 1.003 1.13 1.13 1.134 1.134 10]
      | sbobj.Groups.Signals.YData = [0 0 1 1 0.002 0.002 1 1 0.002 0.002]
  Signal 1 : Outport  Tag=STV Outport
  wires:
  FromWs/1 -> Demux/1
  Demux/1 -> Signal 1/1

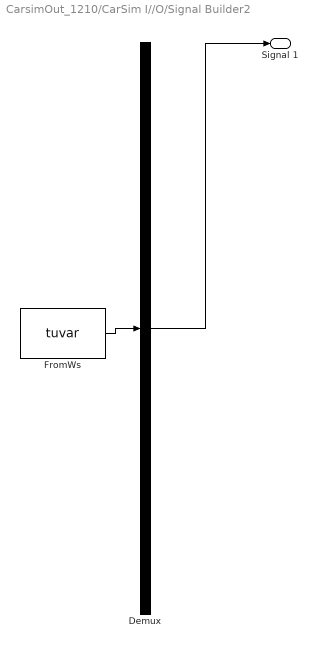
== system CarsimOut_1210/CarSim I//O/Signal Builder2 ==
  Demux : Demux  Tag=STV Demux  Outputs=1
  FromWs : FromWorkspace  Tag=STV FromWs  VariableName=tuvar  SampleTime=0
      SigBuilderData=|
      | common.afterFinalStr = 'Extrapolate'
      | common.sampleTime = 0
      | dataSet.timeRange = [0 10]
      | dataSet.name = 'Group 1'
      | sbobj.Groups.Name = 'Group 1'
      | sbobj.Groups.Signals.Name = 'Signal 1'
      | sbobj.Groups.Signals.XData = [0 4 4 4.003 4.003 4.72 4.72 4.724 4.724 10]
      | sbobj.Groups.Signals.YData = [0 0 1 1 0 0 1 1 0 0]
  Signal 1 : Outport  Tag=STV Outport
  wires:
  Demux/1 -> Signal 1/1
  FromWs/1 -> Demux/1
